simulink model "ip_simulink_main"  (R2015b)
settings: Solver=ode45  StartTime=0.0  StopTime=3  RelTol=1e-5
values from neighbouring files (symbols this model uses):
  A = [0 0 1 0 ... (first row only)    [main.m]
  B = [0 ... (first row only)    [main.m]
  C = [1 0 0 0 ... (first row only)    [main.m]
  K = K_temp    [plots_assignment2.m]    (also in plots_assignment3.m)
settings Model: Creator=magudelo  LastModifiedBy=Mauricio
settings DataIOCC: SaveFormat=Array  SignalLoggingSaveFormat=ModelDataLogs
settings OptimizationCC: ExpressionDepthLimit=2147483647
settings DebuggingCC: UnderspecifiedInitializationDetection=Classic  MergeDetectMultiDrivingBlocksExec=none  SolverPrmCheckMsg=warning  FcnCallInpInsideContextMsg=UseLocalSettings  StateNameClashWarn=warning
settings HardwareCC: ProdBitPerPointer=32  ProdLargestAtomicFloat=None  ProdIntDivRoundTo=Undefined  ProdEndianess=Unspecified  ProdWordSize=32  ProdHWDeviceType=32-bit Generic
settings GRTTargetCC: GeneratePreprocessorConditionals=Disable all  CombineOutputUpdateFcns=off  GRTInterface=on
settings ConfigComp: CovModelRefEnable=Off

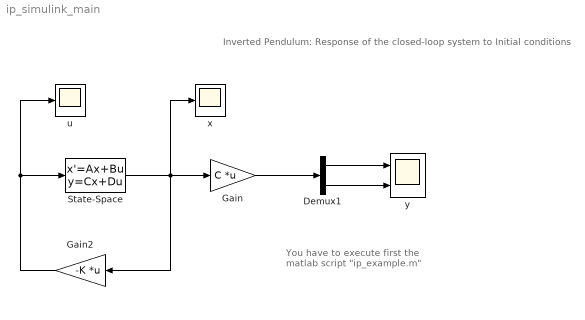
== system ip_simulink_main ==
  note: You have to execute first the
      | matlab script "ip_example.m"
  note: Inverted Pendulum: Response of the closed-loop system to Initial conditions
  Demux1 : Demux  Outputs=2
  Gain : Gain  Gain=C  Multiplication=Matrix(K*u)
  Gain2 : Gain  Gain=-K  Multiplication=Matrix(K*u)
  State-Space : StateSpace  A=A  B=B  C=eye(4)  D=zeros(4,1)  X0=[0 15*pi/180 0 0]
  u : Scope
  x : Scope
  y : Scope  NumInputPorts=2
  wires:
  State-Space/1 -> Gain/1, x/1, Gain2/1
  Gain/1 -> Demux1/1
  Gain2/1 -> u/1, State-Space/1
  Demux1/1 -> y/1
  Demux1/2 -> y/2
